simulink model "a23_all"  (R2014a)
settings: Solver=ode5  StartTime=0.0  StopTime=10.0  FixedStep=0.01  RelTol=1e-3
settings Model: Creator=s65556  LastModifiedBy=s65556

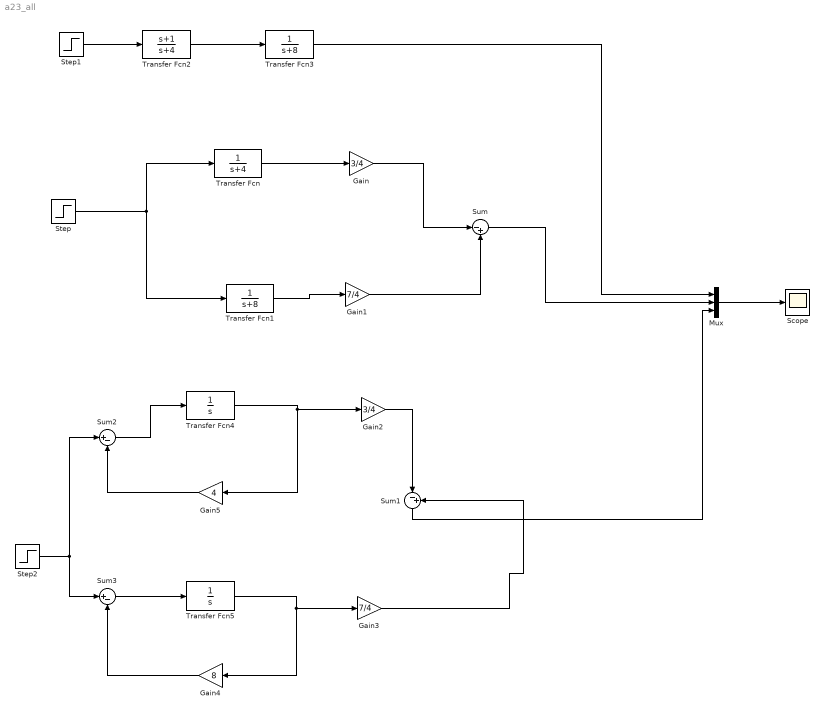
== system a23_all ==
  Gain : Gain  Gain=3/4
  Gain1 : Gain  Gain=7/4
  Gain2 : Gain  Gain=3/4
  Gain3 : Gain  Gain=7/4
  Gain4 : Gain  Gain=8
  Gain5 : Gain  Gain=4
  Mux : Mux  Inputs=3
  Scope : Scope
  Step : Step  SampleTime=0
  Step1 : Step  SampleTime=0
  Step2 : Step  SampleTime=0
  Sum : Sum  Inputs=|-+
  Sum1 : Sum  Inputs=|-+
  Sum2 : Sum  Inputs=|+-
  Sum3 : Sum  Inputs=|+-
  Transfer Fcn : TransferFcn  Denominator=[1 4]
  Transfer Fcn1 : TransferFcn  Denominator=[1 8]
  Transfer Fcn2 : TransferFcn  Numerator=[1 1]  Denominator=[1 4]
  Transfer Fcn3 : TransferFcn  Denominator=[1 8]
  Transfer Fcn4 : TransferFcn  Denominator=[1 0]
  Transfer Fcn5 : TransferFcn  Denominator=[1 0]
  wires:
  Transfer Fcn/1 -> Gain/1
  Gain/1 -> Sum/1
  Step/1 -> Transfer Fcn1/1, Transfer Fcn/1
  Transfer Fcn1/1 -> Gain1/1
  Gain1/1 -> Sum/2
  Step1/1 -> Transfer Fcn2/1
  Transfer Fcn2/1 -> Transfer Fcn3/1
  Step2/1 -> Sum3/1, Sum2/1
  Sum2/1 -> Transfer Fcn4/1
  Transfer Fcn4/1 -> Gain5/1, Gain2/1
  Gain5/1 -> Sum2/2
  Transfer Fcn5/1 -> Gain4/1, Gain3/1
  Gain4/1 -> Sum3/2
  Sum3/1 -> Transfer Fcn5/1
  Gain3/1 -> Sum1/2
  Gain2/1 -> Sum1/1
  Transfer Fcn3/1 -> Mux/1
  Sum/1 -> Mux/2
  Sum1/1 -> Mux/3
  Mux/1 -> Scope/1
